simulink model "H8_6GDL_comparacionNL_Lineal"  (R2022b)
settings: Solver=VariableStepAuto  StartTime=0.0  StopTime=0.45  RelTol=1e-3
InitFcn:
  | lev_nom=0.01965;
values from neighbouring files (symbols this model uses):
  A5 = argout.a    [linealizacion_5gdl_bien.m]    (also in matrices_linealizacion_5gdl.mat = [0 0 0 0 0 0 0 0 0 0 0 0 ... (100 elements, 10x10)])
  B5 = argout.b    [linealizacion_5gdl_bien.m]    (also in matrices_linealizacion_5gdl.mat = [0 0 0 0 0 -0.000575563603666 -0.0459993641186 -0.0506493386)
  C5 = argout.c    [linealizacion_5gdl_bien.m]    (also in matrices_linealizacion_5gdl.mat = [1 0 0 0 0 0 0 0 0 0 0 1 ... (100 elements, 10x10)])
  cg_nom = 0.567    [linealizacion_5gdl.m]    (also in linealizacion_5gdl_bien.m; linealizacion_HEMS.m)
  D5 = argout.d    [linealizacion_5gdl_bien.m]    (also in matrices_linealizacion_5gdl.mat = [0 0 0 0 0 0 0 0 0 0 0 0 ... (80 elements, 10x8)])
settings Model: Creator=aceao  LastModifiedBy=aceao

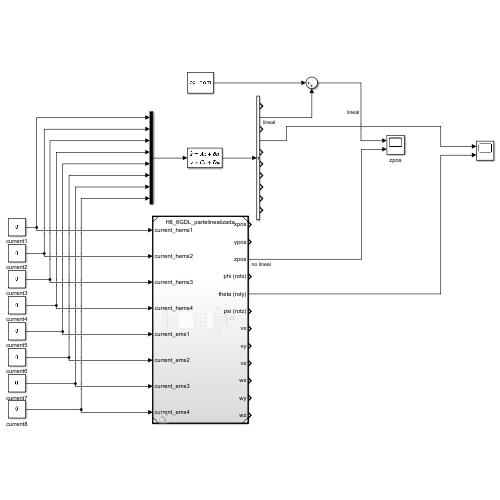
[thumbnail: Simulink's stored preview of the top-level diagram]
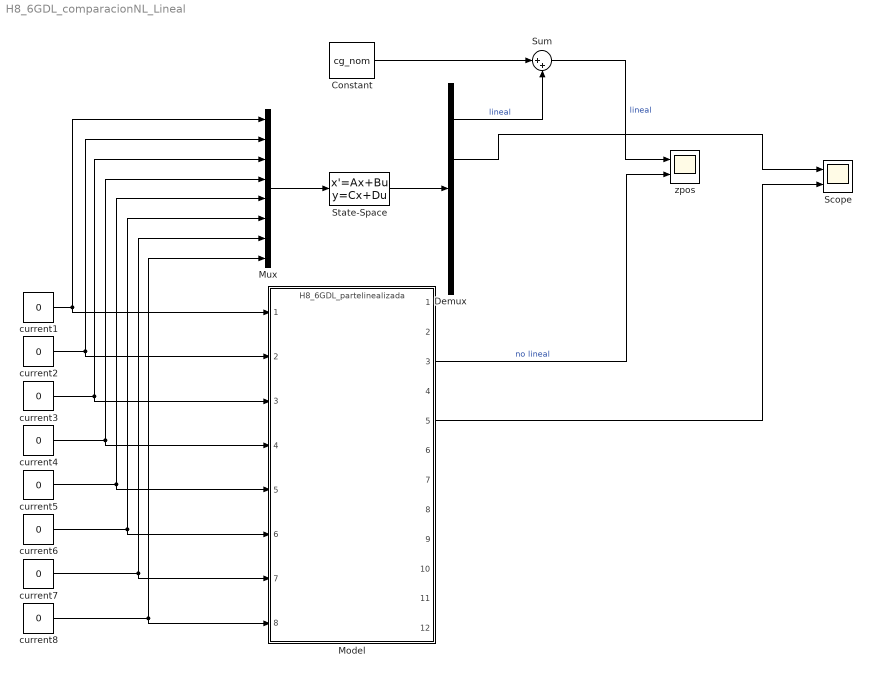
== system H8_6GDL_comparacionNL_Lineal ==
  Constant : Constant  Value=cg_nom
  Demux : Demux  Outputs=10
      settings: DisplayOption=none
  Model : ModelReference  ModelNameDialog=H8_6GDL_partelinealizada.slx  SimulationMode=Normal  ModelReferenceVersion=1.30
  Mux : Mux  Inputs=8
  Scope : Scope  NumInputPorts=2
  State-Space : StateSpace  A=A5  B=B5  C=C5  D=D5  InitialCondition=[0 0.001 0 0 0 0 0 0 0 0]
  Sum : Sum  Inputs=|++
  current{1..8} (8 alike) : Constant  Value=0
  zpos : Scope  NumInputPorts=2
  wires:
  Mux/1 -> State-Space/1
  current1/1 -> Mux/1, Model/1
  current2/1 -> Mux/2, Model/2
  current4/1 -> Mux/4, Model/4
  current3/1 -> Mux/3, Model/3
  current7/1 -> Mux/7, Model/7
  current8/1 -> Mux/8, Model/8
  current6/1 -> Mux/6, Model/6
  current5/1 -> Mux/5, Model/5
  State-Space/1 -> Demux/1
  Constant/1 -> Sum/1
  Sum/1 -> zpos/1  "lineal"
  Demux/2 -> Sum/2  "lineal"
  Model/3 -> zpos/2  "no lineal"
  Demux/4 -> Scope/1
  Model/5 -> Scope/2
